simulink model "model_first_order"  (R2020a)
settings: Solver=VariableStepAuto  StartTime=0.0  StopTime=10.0  RelTol=1e-3
settings Model: Creator=kekatos  LastModifiedBy=kekatos

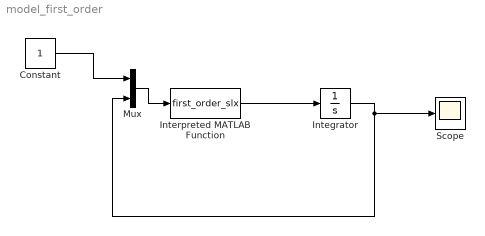
== system model_first_order ==
  Constant : Constant
  Integrator : Integrator  InitialCondition=0.5
  Interpreted MATLAB Function : MATLABFcn  MATLABFcn=first_order_slx
  Mux : Mux  Inputs=2
  Scope : Scope
  wires:
  Constant/1 -> Mux/1
  Mux/1 -> Interpreted MATLAB Function/1
  Interpreted MATLAB Function/1 -> Integrator/1
  Integrator/1 -> Scope/1, Mux/2
